simulink model "Poulin1998"  (R2020b)
settings: Solver=ode4  StartTime=0.0  StopTime=6000  FixedStep=0.01  RelTol=1e-3
values from neighbouring files (symbols this model uses):
  g_f_off = 2.91    [Poulin1998_start.m]
  g_f_on = 2.69    [Poulin1998_start.m]
  g_s = -1.26    [Poulin1998_start.m]
  MCAF_base_on = 99.96    [Poulin1998_start.m]
  PETCO2_base = 40    [Poulin1998_start.m]
  stimHz = stimHzVec(i)    [Poulin1998_start.m]
  tau_f_off = 14.31    [Poulin1998_start.m]
  tau_f_on = 6.77    [Poulin1998_start.m]
  tau_s = 426.9    [Poulin1998_start.m]
  Td = 3.9    [Poulin1998_start.m]
libraries: simulink x1
settings Model: Creator=sider  LastModifiedBy=sider

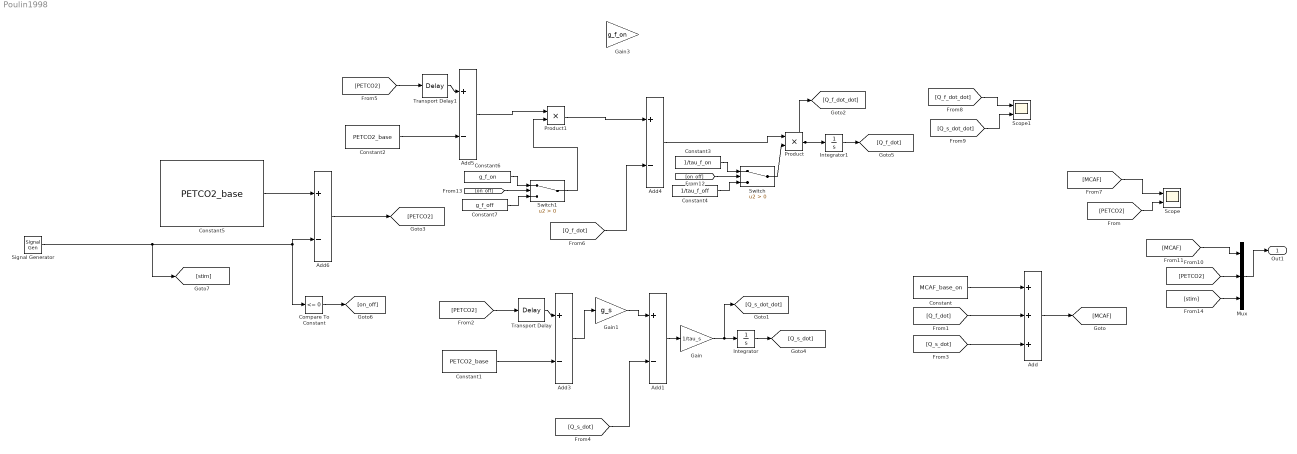
== system Poulin1998 ==
  Add : Sum  Inputs=+++
  Add{1,3..6} (5 alike) : Sum  Inputs=+-
  Compare To Constant : simulink/Logic and Bit Operations/Compare To Constant  relop=<=  const=0  OutDataTypeStr=boolean
  Constant : Constant  Value=MCAF_base_on
  Constant1 : Constant  Value=PETCO2_base
  Constant2 : Constant  Value=PETCO2_base
  Constant3 : Constant  Value=1/tau_f_on
  Constant4 : Constant  Value=1/tau_f_off
  Constant5 : Constant  Value=PETCO2_base
  Constant6 : Constant  Value=g_f_on
  Constant7 : Constant  Value=g_f_off
  Gain : Gain  Gain=1/tau_s
  Gain1 : Gain  Gain=g_s
  Gain3 : Gain  Gain=g_f_on
  Integrator : Integrator
  Integrator1 : Integrator
  Mux : Mux  Inputs=3
  Product : Product
  Product1 : Product
  Scope : Scope  NumInputPorts=2
  Scope1 : Scope  NumInputPorts=2
  Signal Generator : SignalGenerator  Amplitude=2  Frequency=stimHz
  Switch : Switch  Criteria=u2 > Threshold
  Switch1 : Switch  Criteria=u2 > Threshold
  Transport Delay : TransportDelay  DelayTime=Td
  Transport Delay1 : TransportDelay  DelayTime=Td
  Out1 : Outport
  wires:
  Add/1 -> [MCAF]
  Constant/1 -> Add/1
  [Q_f_dot] -> Add/2
  [Q_s_dot] -> Add/3
  Add1/1 -> Gain/1
  Gain/1 -> Integrator/1, [Q_s_dot_dot]
  Gain1/1 -> Add1/1
  [PETCO2] -> Transport Delay/1
  Transport Delay/1 -> Add3/1
  Add3/1 -> Gain1/1
  Constant1/1 -> Add3/2
  [Q_s_dot] -> Add1/2
  Integrator/1 -> [Q_s_dot]
  Product/1 -> [Q_f_dot_dot], Integrator1/1
  Transport Delay1/1 -> Add5/1
  [Q_f_dot] -> Add4/2
  Product1/1 -> Add4/1
  Add5/1 -> Product1/1
  Constant2/1 -> Add5/2
  [PETCO2] -> Transport Delay1/1
  Add4/1 -> Product/1
  Integrator1/1 -> [Q_f_dot]
  [MCAF] -> Scope/1
  [PETCO2] -> Scope/2
  [Q_f_dot_dot] -> Scope1/1
  [Q_s_dot_dot] -> Scope1/2
  Add6/1 -> [PETCO2]
  Constant5/1 -> Add6/1
  Signal Generator/1 -> [stim], Add6/2, Compare To Constant/1
  Mux/1 -> Out1/1
  [MCAF] -> Mux/1
  [PETCO2] -> Mux/2
  Compare To Constant/1 -> [on_off]
  Switch/1 -> Product/2
  [on_off] -> Switch/2
  Constant3/1 -> Switch/1
  Constant4/1 -> Switch/3
  Constant7/1 -> Switch1/3
  Constant6/1 -> Switch1/1
  [on_off] -> Switch1/2
  Switch1/1 -> Product1/2
  [stim] -> Mux/3
